simulink model "ElectricVehicleNMPC"  (R2022b)
settings: Solver=VariableStepAuto  StartTime=0  StopTime=600+N*Ts  RelTol=1e-3
model workspace (MAT data in the model file):
  AccessaryLoad = Simulink.Parameter
  AccessaryLoad.Value = 600
  AccessaryLoad.Description = 'Extra power comsumed in the vehicle.
    | E.g, radio, AC, etc.'
  AccessaryLoad.DataType = 'auto'
  AccessaryLoad.Complexity = 'real'
  AccessaryLoad.Dimensions = [1 1]
  BrakeRegenFraction = Simulink.Parameter
  BrakeRegenFraction.Value = 0.55
  BrakeRegenFraction.DataType = 'auto'
  BrakeRegenFraction.Complexity = 'real'
  BrakeRegenFraction.Dimensions = [1 1]
  Crr = Simulink.Parameter
  Crr.Value = 0.01
  Crr.Description = 'Coefficient of rolling resistence
    | '
  Crr.DataType = 'auto'
  Crr.Complexity = 'real'
  Crr.Dimensions = [1 1]
  DrivelineModelG = Simulink.Parameter
  DrivelineModelG.Value = 3.55
  DrivelineModelG.DataType = 'auto'
  DrivelineModelG.Complexity = 'real'
  DrivelineModelG.Dimensions = [1 1]
  DrivelineModelSpinLoss = Simulink.Parameter
  DrivelineModelSpinLoss.Value = 6
  DrivelineModelSpinLoss.DataType = 'auto'
  DrivelineModelSpinLoss.Complexity = 'real'
  DrivelineModelSpinLoss.Dimensions = [1 1]
  EnergyCapacity = Simulink.Parameter
  EnergyCapacity.Value = 12.6
  EnergyCapacity.Description = 'Energy Capacity of the battery [kWh]'
  EnergyCapacity.DataType = 'auto'
  EnergyCapacity.Complexity = 'real'
  EnergyCapacity.Dimensions = [1 1]
  MassVehInertia = Simulink.Parameter
  MassVehInertia.Value = 2392
  MassVehInertia.Description = 'Inertia of the Vehicle
    | '
  MassVehInertia.DataType = 'auto'
  MassVehInertia.Complexity = 'real'
  MassVehInertia.Dimensions = [1 1]
  MaxPowerOutput = Simulink.Parameter
  MaxPowerOutput.Value = 100000
  MaxPowerOutput.DataType = 'auto'
  MaxPowerOutput.Complexity = 'real'
  MaxPowerOutput.Dimensions = [1 1]
  MaxTorqueOutput = Simulink.Parameter
  MaxTorqueOutput.Value = 500
  MaxTorqueOutput.DataType = 'auto'
  MaxTorqueOutput.Complexity = 'real'
  MaxTorqueOutput.Dimensions = [1 1]
  MaximumBreakForce = Simulink.Parameter
  MaximumBreakForce.Value = 10000
  MaximumBreakForce.Description = 'Maximum Break Force [N]'
  MaximumBreakForce.DataType = 'auto'
  MaximumBreakForce.Complexity = 'real'
  MaximumBreakForce.Dimensions = [1 1]
  MotorModelC = Simulink.Parameter
  MotorModelC.Value = 628.2974
  MotorModelC.DataType = 'auto'
  MotorModelC.Complexity = 'real'
  MotorModelC.Dimensions = [1 1]
  MotorModelKc = Simulink.Parameter
  MotorModelKc.Value = 0.045237
  MotorModelKc.DataType = 'auto'
  MotorModelKc.Complexity = 'real'
  MotorModelKc.Dimensions = [1 1]
  MotorModelKi = Simulink.Parameter
  MotorModelKi.Value = 0.0167
  MotorModelKi.DataType = 'auto'
  MotorModelKi.Complexity = 'real'
  MotorModelKi.Dimensions = [1 1]
  MotorModelKw = Simulink.Parameter
  MotorModelKw.Value = 5.06640055941e-05
  MotorModelKw.DataType = 'auto'
  MotorModelKw.Complexity = 'real'
  MotorModelKw.Dimensions = [1 1]
  N = Simulink.Parameter
  N.Value = 10
  N.Description = 'The number of reference preview for NMPC
    | '
  N.DataType = 'auto'
  N.Complexity = 'real'
  N.Dimensions = [1 1]
  Q = Simulink.Parameter
  Q.Value = 100
  Q.Description = 'Weighting factor of velocity error for cost function
    | '
  Q.DataType = 'auto'
  Q.Complexity = 'real'
  Q.Dimensions = [1 1]
  Rint = Simulink.Parameter
  Rint.Value = 0.1
  Rint.Description = 'Internal Resistence of the battery
    | '
  Rint.DataType = 'auto'
  Rint.Complexity = 'real'
  Rint.Dimensions = [1 1]
  Ts = Simulink.Parameter
  Ts.Value = 0.01
  Ts.Description = 'Sample Time'
  Ts.DataType = 'auto'
  Ts.Complexity = 'real'
  Ts.Dimensions = [1 1]
  Voc = Simulink.Parameter
  Voc.Value = 340
  Voc.Description = 'Open Circuit Voltage of the Battery'
  Voc.DataType = 'auto'
  Voc.Complexity = 'real'
  Voc.Dimensions = [1 1]
  gravity = Simulink.Parameter
  gravity.Value = 9.81
  gravity.Description = 'Gravity constant
    | '
  gravity.DataType = 'auto'
  gravity.Complexity = 'real'
  gravity.Dimensions = [1 1]
  massVeh = Simulink.Parameter
  massVeh.Value = 2300
  massVeh.Description = 'Vehicle Mass
    | '
  massVeh.DataType = 'auto'
  massVeh.DocUnits = 'kg'
  massVeh.Complexity = 'real'
  massVeh.Dimensions = [1 1]
  theta = Simulink.Parameter
  theta.Value = 0
  theta.Description = 'Road Grade
    | '
  theta.DataType = 'auto'
  theta.DocUnits = 'radian'
  theta.Complexity = 'real'
  theta.Dimensions = [1 1]
  wheelRadius = Simulink.Parameter
  wheelRadius.Value = 0.34
  wheelRadius.Description = 'meter'
  wheelRadius.DataType = 'auto'
  wheelRadius.Complexity = 'real'
  wheelRadius.Dimensions = [1 1]
values from neighbouring files (symbols this model uses):
  AccessaryLoad = 600    [NMPC_EV.m]
  BrakeRegenFraction = 0.55    [NMPC_EV.m]
  Crr = 0.01    [NMPC_EV.m]
  DrivelineModelG = 3.55    [NMPC_EV.m]
  DrivelineModelSpinLoss = 6    [NMPC_EV.m]
  EnergyCapacity = 12.6    [NMPC_EV.m]
  gravity = 9.81    [NMPC_EV.m]
  m = 2    [NMPC_EV.m]
  massVeh = 2300    [NMPC_EV.m]
  MassVehInertia = 2392    [NMPC_EV.m]
  MaximumBreakForce = 10000    [NMPC_EV.m]
  MaxPowerOutput = 1e5    (= 100000)    [NMPC_EV.m]
  MaxTorqueOutput = 500    [NMPC_EV.m]
  MotorModelC = 628.2974    [NMPC_EV.m]
  MotorModelKc = 0.045237    [NMPC_EV.m]
  MotorModelKi = 0.0167    [NMPC_EV.m]
  MotorModelKw = 5.06640055940796E-5    (= 5.06640055941e-05)    [NMPC_EV.m]
  N = 5    [NMPC_EV.m]
  Q = 3000    [NMPC_EV.m]
  Rint = 0.1    [NMPC_EV.m]
  Ts = 0.01    [NMPC_EV.m]
  Voc = 340    [NMPC_EV.m]
  wheelRadius = 0.34    [NMPC_EV.m]
libraries: simulink x12, autolibshared x2
(part 1 of 2)
settings Model: SimulationMode=accelerator  Creator=allen  LastModifiedBy=allen

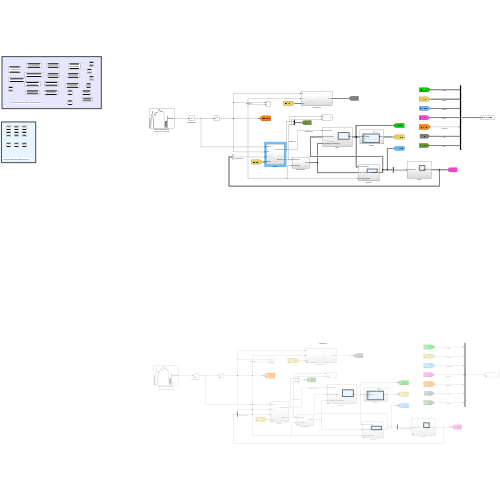
[thumbnail: Simulink's stored preview of the top-level diagram]
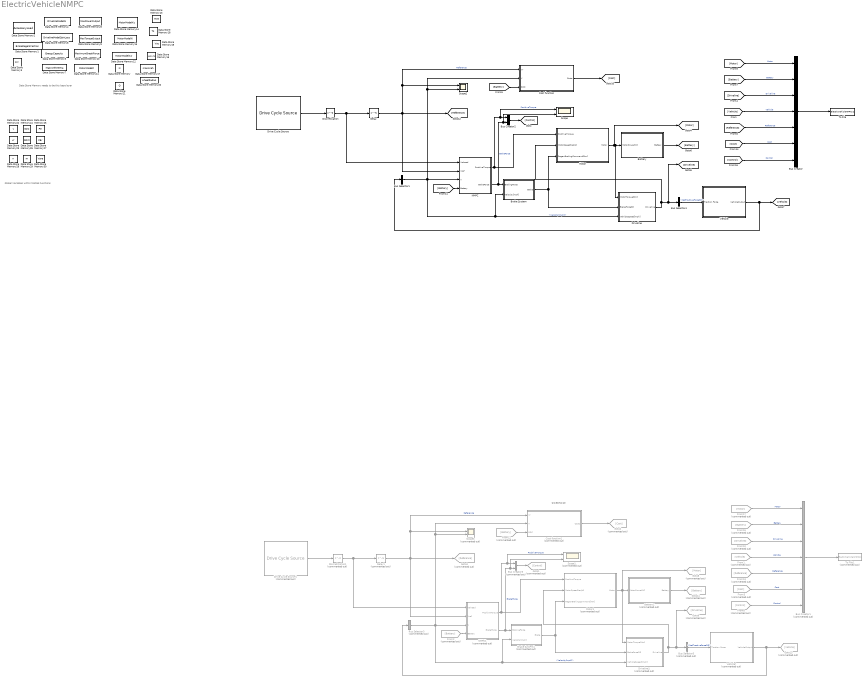
== system ElectricVehicleNMPC ==
  note: Q=30;N=10
  note: Global Variables within Matlab Functions
  note: Data Store Memory needs to be this base layer
  Battery : Subsystem
  Battery1 : Subsystem  Commented=on
  Brake System : Subsystem
  Brake System1 : Subsystem  Commented=on
  Bus Creator : BusCreator  Inputs=7
  Bus Creator1 : BusCreator  Commented=on  Inputs=7
  Bus Creator2 : BusCreator  Inputs=2
  Bus Creator3 : BusCreator  Commented=on  Inputs=2
  Bus Selector1 : BusSelector  OutputSignals=Velocity[mph]
  Bus Selector3 : BusSelector  Commented=on  OutputSignals=Velocity[mph]
  Bus Selector4 : BusSelector  OutputSignals=NetTractiveForce[N]
  Bus Selector5 : BusSelector  Commented=on  OutputSignals=NetTractiveForce[N]
  Cost function : Subsystem
  Cost function1 : Subsystem  Commented=on
  Data Store Memory : DataStoreMemory  DataStoreName=N  WriteAfterWriteMsg=warning  InitialValue=N  ShowAdditionalParam=off  OutDataTypeStr=double
  Data Store Memory1 : DataStoreMemory  DataStoreName=BrakeRegenFraction  WriteAfterWriteMsg=warning  InitialValue=BrakeRegenFraction  ShowAdditionalParam=off  OutDataTypeStr=double
  Data Store Memory10 : DataStoreMemory  DataStoreName=MaximumBreakForce  WriteAfterWriteMsg=warning  InitialValue=MaximumBreakForce  ShowAdditionalParam=off  OutDataTypeStr=double
  Data Store Memory11 : DataStoreMemory  DataStoreName=MotorModelC  WriteAfterWriteMsg=warning  InitialValue=MotorModelC  ShowAdditionalParam=off  OutDataTypeStr=double
  Data Store Memory12 : DataStoreMemory  DataStoreName=MotorModelKw  WriteAfterWriteMsg=warning  InitialValue=MotorModelKw  ShowAdditionalParam=off  OutDataTypeStr=double
  Data Store Memory13 : DataStoreMemory  DataStoreName=Rint  WriteAfterWriteMsg=warning  InitialValue=Rint  ShowAdditionalParam=off  OutDataTypeStr=double
  Data Store Memory14 : DataStoreMemory  DataStoreName=MotorModelKc  WriteAfterWriteMsg=warning  InitialValue=MotorModelKc  ShowAdditionalParam=off  OutDataTypeStr=double
  Data Store Memory15 : DataStoreMemory  DataStoreName=MotorModelKi  WriteAfterWriteMsg=warning  InitialValue=MotorModelKi  ShowAdditionalParam=off  OutDataTypeStr=double
  Data Store Memory16 : DataStoreMemory  DataStoreName=gravity  WriteAfterWriteMsg=warning  InitialValue=gravity  ShowAdditionalParam=off  OutDataTypeStr=double
  Data Store Memory17 : DataStoreMemory  DataStoreName=massVeh  WriteAfterWriteMsg=warning  InitialValue=massVeh  ShowAdditionalParam=off  OutDataTypeStr=double
  Data Store Memory18 : DataStoreMemory  DataStoreName=Ts  WriteAfterWriteMsg=warning  InitialValue=Ts  ShowAdditionalParam=off  OutDataTypeStr=double
  Data Store Memory19 : DataStoreMemory  DataStoreName=Voc  WriteAfterWriteMsg=warning  InitialValue=Voc  ShowAdditionalParam=off  OutDataTypeStr=double
  Data Store Memory2 : DataStoreMemory  DataStoreName=AccessaryLoad  WriteAfterWriteMsg=warning  InitialValue=AccessaryLoad  ShowAdditionalParam=off  OutDataTypeStr=double
  Data Store Memory20 : DataStoreMemory  DataStoreName=wheelRadius  WriteAfterWriteMsg=warning  InitialValue=wheelRadius  ShowAdditionalParam=off  OutDataTypeStr=double
  Data Store Memory21 : DataStoreMemory  DataStoreName=Q  WriteAfterWriteMsg=warning  InitialValue=Q  ShowAdditionalParam=off  OutDataTypeStr=double
  Data Store Memory22 : DataStoreMemory  DataStoreName=v  WriteAfterWriteMsg=warning  ShowAdditionalParam=off  OutDataTypeStr=double
  Data Store Memory23 : DataStoreMemory  DataStoreName=vr  WriteAfterWriteMsg=warning  ShowAdditionalParam=off  OutDataTypeStr=double
  Data Store Memory24 : DataStoreMemory  DataStoreName=SOC  WriteAfterWriteMsg=warning  ShowAdditionalParam=off  OutDataTypeStr=double
  Data Store Memory25 : DataStoreMemory  DataStoreName=Ptr  WriteAfterWriteMsg=warning  ShowAdditionalParam=off  OutDataTypeStr=double  Dimensions=[N+1,1]
  Data Store Memory26 : DataStoreMemory  DataStoreName=SOCr  WriteAfterWriteMsg=warning  InitialValue=100  ShowAdditionalParam=off  OutDataTypeStr=double
  Data Store Memory27 : DataStoreMemory  DataStoreName=FBr  WriteAfterWriteMsg=warning  ShowAdditionalParam=off  OutDataTypeStr=double  Dimensions=[N+1,1]
  Data Store Memory28 : DataStoreMemory  DataStoreName=n  WriteAfterWriteMsg=warning  InitialValue=2  ShowAdditionalParam=off  OutDataTypeStr=double
  Data Store Memory29 : DataStoreMemory  DataStoreName=m  WriteAfterWriteMsg=warning  InitialValue=2  ShowAdditionalParam=off  OutDataTypeStr=double
  Data Store Memory3 : DataStoreMemory  DataStoreName=Crr  WriteAfterWriteMsg=warning  InitialValue=Crr  ShowAdditionalParam=off  OutDataTypeStr=double
  Data Store Memory30 : DataStoreMemory  DataStoreName=Vpre  WriteAfterWriteMsg=warning  ShowAdditionalParam=off  OutDataTypeStr=double  Dimensions=[N+1,1]
  Data Store Memory4 : DataStoreMemory  DataStoreName=DrivelineModelG  WriteAfterWriteMsg=warning  InitialValue=DrivelineModelG  ShowAdditionalParam=off  OutDataTypeStr=double
  Data Store Memory5 : DataStoreMemory  DataStoreName=EnergyCapacity  WriteAfterWriteMsg=warning  InitialValue=EnergyCapacity  ShowAdditionalParam=off  OutDataTypeStr=double
  Data Store Memory6 : DataStoreMemory  DataStoreName=DrivelineModelSpinLoss  WriteAfterWriteMsg=warning  InitialValue=DrivelineModelSpinLoss  ShowAdditionalParam=off  OutDataTypeStr=double
  Data Store Memory7 : DataStoreMemory  DataStoreName=MassVehInertia  WriteAfterWriteMsg=warning  InitialValue=MassVehInertia  ShowAdditionalParam=off  OutDataTypeStr=double
  Data Store Memory8 : DataStoreMemory  DataStoreName=MaxPowerOutput  WriteAfterWriteMsg=warning  InitialValue=MaxPowerOutput  ShowAdditionalParam=off  OutDataTypeStr=double
  Data Store Memory9 : DataStoreMemory  DataStoreName=MaxTorqueOutput  WriteAfterWriteMsg=warning  InitialValue=MaxTorqueOutput  ShowAdditionalParam=off  OutDataTypeStr=double
  Delay : Delay  DelayLength=N
  Delay1 : Delay  Commented=on  DelayLength=N
  Discretization : Delay  DelayLength=0  SampleTime=Ts
  Discretization1 : Delay  Commented=on  DelayLength=0  SampleTime=Ts
  Drive Cycle Source : autolibshared/Drive Cycle Source  cycleVar=US06  fileVar=cycleFTP75.mat  tfinal="600  seconds"  cycleRepeat=off  outAccPort=off  outGearPort=off  gearList=No gear data  t_wot1=5  xdot_woto=0  xdot_wot1=30  t_wot2=20  xdot_wot2=0  t_wotend=30  srcUnit=m/s  outUnit=mph  srcAccUnit=m/s/s  outAccUnit=m/s^2  dt=0  aMode=1  faultOption=off  velBnd=2  velBndUnit=mph  inUnit=m/s  timeBnd=1  failOption=off  stopSim=off  maxFaultCnt=10  maxFaultTime=2  maxTotFaultTime=15  traceOption=off  dtTrace=1  traceWindow=10  lastDCname=US06  lastOutUnit=mph  lastDT=0  lastTB=1  lastSB=2  forceCalcBound=off
  Drive Cycle Source1 : autolibshared/Drive Cycle Source  Commented=on  cycleVar=US06  fileVar=cycleFTP75.mat  tfinal="600  seconds"  cycleRepeat=off  outAccPort=off  outGearPort=off  gearList=No gear data  t_wot1=5  xdot_woto=0  xdot_wot1=30  t_wot2=20  xdot_wot2=0  t_wotend=30  srcUnit=m/s  outUnit=mph  srcAccUnit=m/s/s  outAccUnit=m/s^2  dt=0  aMode=1  faultOption=off  velBnd=2  velBndUnit=mph  inUnit=m/s  timeBnd=1  failOption=off  stopSim=off  maxFaultCnt=10  maxFaultTime=2  maxTotFaultTime=15  traceOption=off  dtTrace=1  traceWindow=10  lastDCname=US06  lastOutUnit=mph  lastDT=0  lastTB=1  lastSB=2  forceCalcBound=off
  Driveline : Subsystem
  Driveline1 : Subsystem  Commented=on
  From1 : From  Commented=on  GotoTag=Vehicle
  From10 : From  Commented=on  GotoTag=Driveline
  From12 : From  Commented=on  GotoTag=Battery
  From13 : From  Commented=on  GotoTag=Reference
  From15 : From  Commented=on  GotoTag=Battery
  From17 : From  Commented=on  GotoTag=Motor
  From2 : From  Commented=on  GotoTag=Battery
  From3 : From  Commented=on  GotoTag=Cost
  From8 : From  Commented=on  GotoTag=Control
  Goto1 : Goto  Commented=on  GotoTag=Control
  Goto11 : Goto  Commented=on  GotoTag=Battery
  Goto13 : Goto  Commented=on  GotoTag=Vehicle
  Goto2 : Goto  Commented=on  GotoTag=Cost
  Goto3 : Goto  Commented=on  GotoTag=Reference
  Goto8 : Goto  Commented=on  GotoTag=Motor
  Goto9 : Goto  Commented=on  GotoTag=Driveline
  Motor : Subsystem
  Motor1 : Subsystem  Commented=on
  NMPC : Subsystem
  NMPC1 : Subsystem  Commented=on
  Scope : Scope  NumInputPorts=2
  Scope1 : Scope  Commented=on  NumInputPorts=2
  Scope2 : Scope  NumInputPorts=2
  Scope3 : Scope  Commented=on  NumInputPorts=2
  To File : ToFile  Filename=ElectricVehicleNMPCv2  MatrixName=Data  SaveFormat=Timeseries
  To File1 : ToFile  Commented=on  Filename=ElectricVehicleNMPC1k  MatrixName=Data  SaveFormat=Timeseries
  Vehicle : Subsystem
  Vehicle1 : Subsystem  Commented=on
  wires:
  Motor/1(Motor) -> [Motor], Driveline/1(MotorTorque[Nm]), Battery/1(MotorPower[W])
  Bus Selector1/1 -> Brake System/2(Velocity[mph]), Driveline/3(VehicleSpeed[mph]), Scope2/2, Cost function/2(V), NMPC/3(V)  "<Velocity[mph]>"
  Driveline/1(Driveline) -> Motor/2(MotorSpeed[rad/s]), [Driveline], Bus Selector4/1
  Drive Cycle Source/1 -> Discretization/1
  Bus Selector4/1 -> Vehicle/1(Traction Force)  "<NetTractiveForce[N]>"
  Battery/1(Battery) -> [Battery]
  Vehicle/1(VehicleOutput) -> [Vehicle], Bus Selector1/1
  [Battery] -> Cost function/3(SOC)
  Brake System/1(Brake) -> Motor/3(RegenBrakingCommand[Nm]), Driveline/2(BrakeForce[N])
  NMPC/1(PositiveTorque) -> Scope/1, Bus Creator2/1, Motor/1(PositiveTorque)  "PositiveTorque"
  NMPC/2(BrakeForce) -> Scope/2, Bus Creator2/2, Brake System/1(BrakingForce)  "BrakeForce"
  [Battery] -> NMPC/4(Battery)
  Delay/1 -> [Reference], NMPC/2(Vref), Scope2/1, Cost function/1(Vr)  "Reference"
  Discretization/1 -> NMPC/1(Vahead), Delay/1
  Bus Creator/1 -> To File/1
  [Driveline] -> Bus Creator/3  "Driveline"
  [Reference] -> Bus Creator/5  "Reference"
  [Cost] -> Bus Creator/6  "Cost"
  [Vehicle] -> Bus Creator/4  "Vehicle"
  [Motor] -> Bus Creator/1  "Motor"
  [Battery] -> Bus Creator/2  "Battery"
  Cost function/1(Costs) -> [Cost]
  Bus Creator2/1 -> [Control]
  [Control] -> Bus Creator/7  "Control"
  Battery1/1(Battery) -> Goto11/1
  Driveline1/1(Driveline) -> Motor1/2(MotorSpeed[rad/s]), Goto9/1, Bus Selector5/1
  Bus Selector5/1 -> Vehicle1/1(Traction Force)  "<NetTractiveForce[N]>"
  Delay1/1 -> Goto3/1, NMPC1/2(Vref), Scope3/1, Cost function1/1(Vr)  "Reference"
  From8/1 -> Bus Creator1/7  "Control"
  NMPC1/1(PositiveTorque) -> Scope1/1, Bus Creator3/1, Motor1/1(PositiveTorque)  "PositiveTorque"
  From1/1 -> Bus Creator1/4  "Vehicle"
  Bus Creator3/1 -> Goto1/1
  From15/1 -> Bus Creator1/2  "Battery"
  Bus Selector3/1 -> Brake System1/2(Velocity[mph]), Driveline1/3(VehicleSpeed[mph]), Scope3/2, Cost function1/2(V), NMPC1/3(V)  "<Velocity[mph]>"
  From12/1 -> Cost function1/3(SOC)
  NMPC1/2(BrakeForce) -> Scope1/2, Bus Creator3/2, Brake System1/1(BrakingForce)  "BrakeForce"
  From2/1 -> NMPC1/4(Battery)
  Discretization1/1 -> NMPC1/1(Vahead), Delay1/1
  From13/1 -> Bus Creator1/5  "Reference"
  From3/1 -> Bus Creator1/6  "Cost"
  Bus Creator1/1 -> To File1/1
  From10/1 -> Bus Creator1/3  "Driveline"
  Cost function1/1(Costs) -> Goto2/1
  Vehicle1/1(VehicleOutput) -> Goto13/1, Bus Selector3/1
  From17/1 -> Bus Creator1/1  "Motor"
  Motor1/1(Motor) -> Goto8/1, Driveline1/1(MotorTorque[Nm]), Battery1/1(MotorPower[W])
  Drive Cycle Source1/1 -> Discretization1/1
  Brake System1/1(Brake) -> Motor1/3(RegenBrakingCommand[Nm]), Driveline1/2(BrakeForce[N])

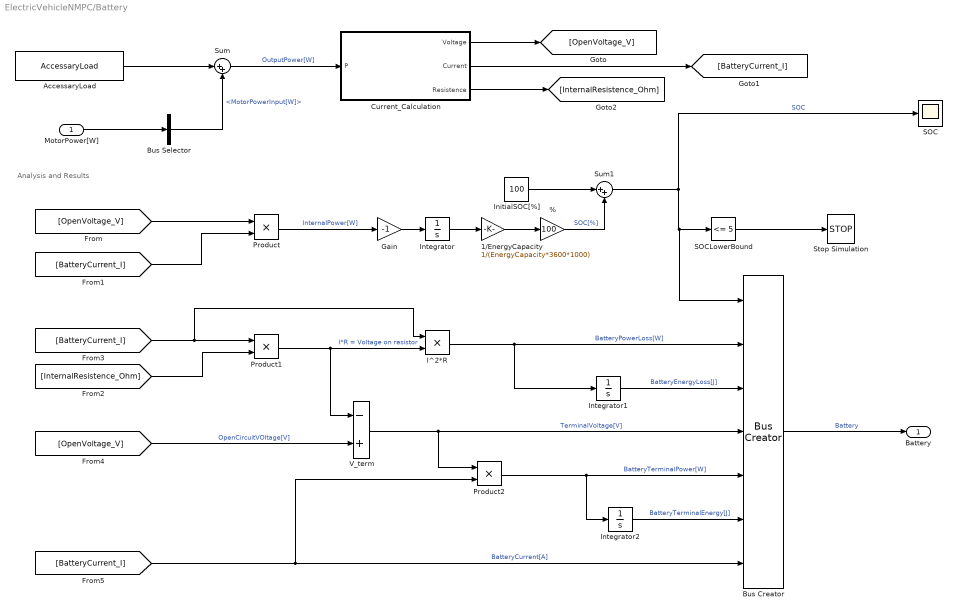
== system ElectricVehicleNMPC/Battery ==
  note: Analysis and Results
  MotorPower[W] : Inport
  % : Gain  Gain=100
  1/EnergyCapacity : Gain  Gain=1/(EnergyCapacity*3600*1000)
  AccessaryLoad : Constant  Value=AccessaryLoad
  Bus Creator : BusCreator  Inputs=7
  Bus Selector : BusSelector  OutputSignals=MotorPowerInput[W]
  Current_Calculation : Subsystem
  Gain : Gain  Gain=-1
  I^2*R : Product
  InitialSOC[%] : Constant  Value=100
  Integrator : Integrator
  Integrator1 : Integrator
  Integrator2 : Integrator
  Product : Product
  Product1 : Product
  Product2 : Product
  SOC : Scope
  SOCLowerBound : simulink/Logic and Bit Operations/Compare To Constant  relop=<=  const=5  OutDataTypeStr=boolean
  Stop Simulation : Stop
  Sum : Sum  Inputs=|++
  Sum1 : Sum  Inputs=|++
  V_term : Sum  Inputs=-+
  Battery : Outport
  wires:
  AccessaryLoad/1 -> Sum/1
  Sum/1 -> Current_Calculation/1(P)  "OutputPower[W]"
  MotorPower[W]/1 -> Bus Selector/1
  Current_Calculation/1(Voltage) -> [OpenVoltage_V]
  Current_Calculation/2(Current) -> [BatteryCurrent_I]
  Current_Calculation/3(Resistence) -> [InternalResistence_Ohm]
  [OpenVoltage_V] -> Product/1
  [BatteryCurrent_I] -> Product/2
  Product/1 -> Gain/1  "InternalPower[W]"
  Gain/1 -> Integrator/1
  Integrator/1 -> 1/EnergyCapacity/1
  1/EnergyCapacity/1 -> %/1
  %/1 -> Sum1/2  "SOC[%]"
  SOCLowerBound/1 -> Stop Simulation/1
  [BatteryCurrent_I] -> I^2*R/1, Product1/1
  [InternalResistence_Ohm] -> Product1/2
  Product1/1 -> V_term/1, I^2*R/2  "I*R = Voltage on resistor"
  I^2*R/1 -> Integrator1/1, Bus Creator/2  "BatteryPowerLoss[W]"
  Integrator1/1 -> Bus Creator/3  "BatteryEnergyLoss[J]"
  [OpenVoltage_V] -> V_term/2  "OpenCircuitVOltage[V]"
  V_term/1 -> Product2/1, Bus Creator/4  "TerminalVoltage[V]"
  [BatteryCurrent_I] -> Product2/2, Bus Creator/7  "BatteryCurrent[A]"
  Product2/1 -> Integrator2/1, Bus Creator/5  "BatteryTerminalPower[W]"
  Integrator2/1 -> Bus Creator/6  "BatteryTerminalEnergy[J]"
  Bus Creator/1 -> Battery/1  "Battery"
  Bus Selector/1 -> Sum/2  "<MotorPowerInput[W]>"
  InitialSOC[%]/1 -> Sum1/1
  Sum1/1 -> Bus Creator/1, SOCLowerBound/1, SOC/1  "SOC"

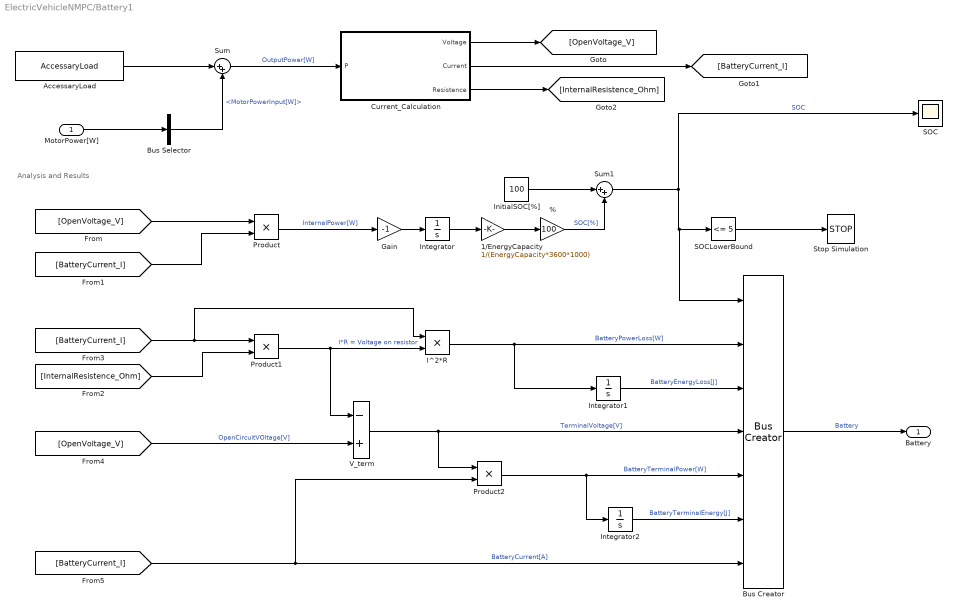
== system ElectricVehicleNMPC/Battery1 ==
  note: Analysis and Results
  MotorPower[W] : Inport
  % : Gain  Gain=100
  1/EnergyCapacity : Gain  Gain=1/(EnergyCapacity*3600*1000)
  AccessaryLoad : Constant  Value=AccessaryLoad
  Bus Creator : BusCreator  Inputs=7
  Bus Selector : BusSelector  OutputSignals=MotorPowerInput[W]
  Current_Calculation : Subsystem
  Gain : Gain  Gain=-1
  I^2*R : Product
  InitialSOC[%] : Constant  Value=100
  Integrator : Integrator
  Integrator1 : Integrator
  Integrator2 : Integrator
  Product : Product
  Product1 : Product
  Product2 : Product
  SOC : Scope
  SOCLowerBound : simulink/Logic and Bit Operations/Compare To Constant  relop=<=  const=5  OutDataTypeStr=boolean
  Stop Simulation : Stop
  Sum : Sum  Inputs=|++
  Sum1 : Sum  Inputs=|++
  V_term : Sum  Inputs=-+
  Battery : Outport
  wires:
  AccessaryLoad/1 -> Sum/1
  Sum/1 -> Current_Calculation/1(P)  "OutputPower[W]"
  MotorPower[W]/1 -> Bus Selector/1
  Current_Calculation/1(Voltage) -> [OpenVoltage_V]
  Current_Calculation/2(Current) -> [BatteryCurrent_I]
  Current_Calculation/3(Resistence) -> [InternalResistence_Ohm]
  [OpenVoltage_V] -> Product/1
  [BatteryCurrent_I] -> Product/2
  Product/1 -> Gain/1  "InternalPower[W]"
  Gain/1 -> Integrator/1
  Integrator/1 -> 1/EnergyCapacity/1
  1/EnergyCapacity/1 -> %/1
  %/1 -> Sum1/2  "SOC[%]"
  SOCLowerBound/1 -> Stop Simulation/1
  [BatteryCurrent_I] -> I^2*R/1, Product1/1
  [InternalResistence_Ohm] -> Product1/2
  Product1/1 -> V_term/1, I^2*R/2  "I*R = Voltage on resistor"
  I^2*R/1 -> Integrator1/1, Bus Creator/2  "BatteryPowerLoss[W]"
  Integrator1/1 -> Bus Creator/3  "BatteryEnergyLoss[J]"
  [OpenVoltage_V] -> V_term/2  "OpenCircuitVOltage[V]"
  V_term/1 -> Product2/1, Bus Creator/4  "TerminalVoltage[V]"
  [BatteryCurrent_I] -> Product2/2, Bus Creator/7  "BatteryCurrent[A]"
  Product2/1 -> Integrator2/1, Bus Creator/5  "BatteryTerminalPower[W]"
  Integrator2/1 -> Bus Creator/6  "BatteryTerminalEnergy[J]"
  Bus Creator/1 -> Battery/1  "Battery"
  Bus Selector/1 -> Sum/2  "<MotorPowerInput[W]>"
  InitialSOC[%]/1 -> Sum1/1
  Sum1/1 -> Bus Creator/1, SOCLowerBound/1, SOC/1  "SOC"

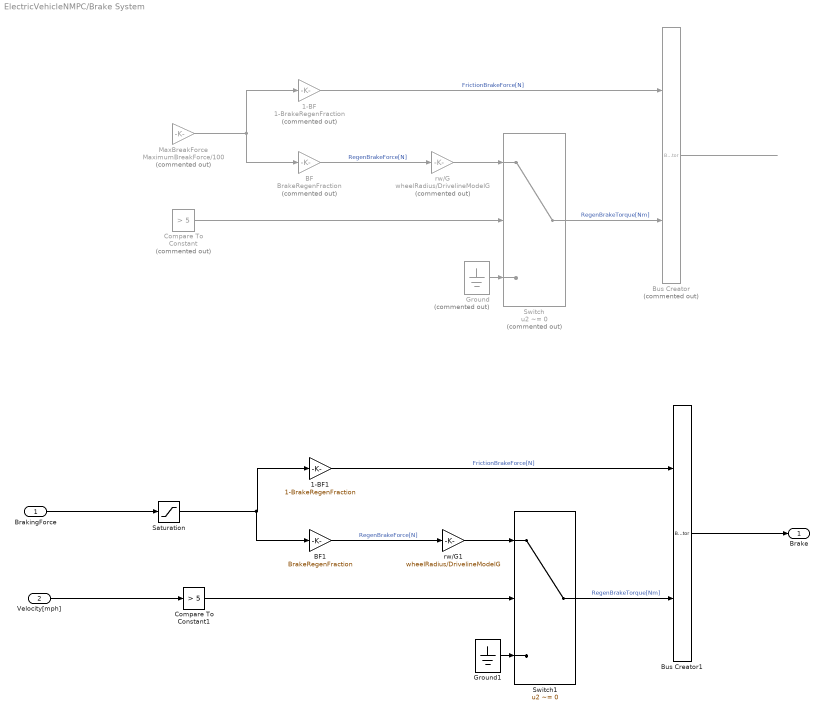
== system ElectricVehicleNMPC/Brake System ==
  BrakingForce : Inport
  Velocity[mph] : Inport  Port=2
  1-BF : Gain  Commented=on  Gain=1-BrakeRegenFraction
  1-BF1 : Gain  Gain=1-BrakeRegenFraction
  BF : Gain  Commented=on  Gain=BrakeRegenFraction
  BF1 : Gain  Gain=BrakeRegenFraction
  Bus Creator : BusCreator  Commented=on  Inputs=2
  Bus Creator1 : BusCreator  Inputs=2
  Compare To Constant : simulink/Logic and Bit Operations/Compare To Constant  Commented=on  relop=>  const=5  OutDataTypeStr=boolean
  Compare To Constant1 : simulink/Logic and Bit Operations/Compare To Constant  relop=>  const=5  OutDataTypeStr=boolean
  Ground : Ground  Commented=on
  Ground1 : Ground
  MaxBreakForce : Gain  Commented=on  Gain=MaximumBreakForce/100
  Saturation : Saturate  UpperLimit=0  LowerLimit=-MaximumBreakForce
  Switch : Switch  Commented=on  Criteria=u2 ~= 0  SaturateOnIntegerOverflow=off  InputSameDT=off
  Switch1 : Switch  Criteria=u2 ~= 0  SaturateOnIntegerOverflow=off  InputSameDT=off
  rw/G : Gain  Commented=on  Gain=wheelRadius/DrivelineModelG
  rw/G1 : Gain  Gain=wheelRadius/DrivelineModelG
  Brake : Outport
  wires:
  Compare To Constant/1 -> Switch/2
  Ground/1 -> Switch/3
  MaxBreakForce/1 -> BF/1, 1-BF/1
  BF/1 -> rw/G/1  "RegenBrakeForce[N]"
  rw/G/1 -> Switch/1
  Switch/1 -> Bus Creator/2  "RegenBrakeTorque[Nm]"
  1-BF/1 -> Bus Creator/1  "FrictionBrakeForce[N]"
  Bus Creator/1 -> ?
  Ground1/1 -> Switch1/3
  rw/G1/1 -> Switch1/1
  Switch1/1 -> Bus Creator1/2  "RegenBrakeTorque[Nm]"
  Bus Creator1/1 -> Brake/1
  Velocity[mph]/1 -> Compare To Constant1/1
  1-BF1/1 -> Bus Creator1/1  "FrictionBrakeForce[N]"
  BF1/1 -> rw/G1/1  "RegenBrakeForce[N]"
  BrakingForce/1 -> Saturation/1
  Compare To Constant1/1 -> Switch1/2
  Saturation/1 -> BF1/1, 1-BF1/1

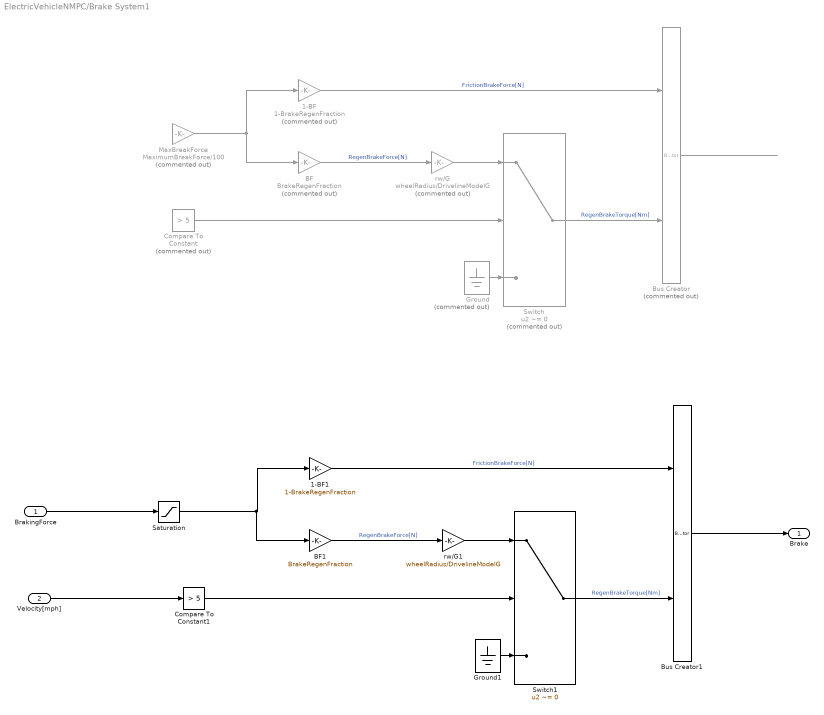
== system ElectricVehicleNMPC/Brake System1 ==
  BrakingForce : Inport
  Velocity[mph] : Inport  Port=2
  1-BF : Gain  Commented=on  Gain=1-BrakeRegenFraction
  1-BF1 : Gain  Gain=1-BrakeRegenFraction
  BF : Gain  Commented=on  Gain=BrakeRegenFraction
  BF1 : Gain  Gain=BrakeRegenFraction
  Bus Creator : BusCreator  Commented=on  Inputs=2
  Bus Creator1 : BusCreator  Inputs=2
  Compare To Constant : simulink/Logic and Bit Operations/Compare To Constant  Commented=on  relop=>  const=5  OutDataTypeStr=boolean
  Compare To Constant1 : simulink/Logic and Bit Operations/Compare To Constant  relop=>  const=5  OutDataTypeStr=boolean
  Ground : Ground  Commented=on
  Ground1 : Ground
  MaxBreakForce : Gain  Commented=on  Gain=MaximumBreakForce/100
  Saturation : Saturate  UpperLimit=0  LowerLimit=-MaximumBreakForce
  Switch : Switch  Commented=on  Criteria=u2 ~= 0  SaturateOnIntegerOverflow=off  InputSameDT=off
  Switch1 : Switch  Criteria=u2 ~= 0  SaturateOnIntegerOverflow=off  InputSameDT=off
  rw/G : Gain  Commented=on  Gain=wheelRadius/DrivelineModelG
  rw/G1 : Gain  Gain=wheelRadius/DrivelineModelG
  Brake : Outport
  wires:
  Compare To Constant/1 -> Switch/2
  Ground/1 -> Switch/3
  MaxBreakForce/1 -> BF/1, 1-BF/1
  BF/1 -> rw/G/1  "RegenBrakeForce[N]"
  rw/G/1 -> Switch/1
  Switch/1 -> Bus Creator/2  "RegenBrakeTorque[Nm]"
  1-BF/1 -> Bus Creator/1  "FrictionBrakeForce[N]"
  Bus Creator/1 -> ?
  Ground1/1 -> Switch1/3
  rw/G1/1 -> Switch1/1
  Switch1/1 -> Bus Creator1/2  "RegenBrakeTorque[Nm]"
  Bus Creator1/1 -> Brake/1
  Velocity[mph]/1 -> Compare To Constant1/1
  1-BF1/1 -> Bus Creator1/1  "FrictionBrakeForce[N]"
  BF1/1 -> rw/G1/1  "RegenBrakeForce[N]"
  BrakingForce/1 -> Saturation/1
  Compare To Constant1/1 -> Switch1/2
  Saturation/1 -> BF1/1, 1-BF1/1

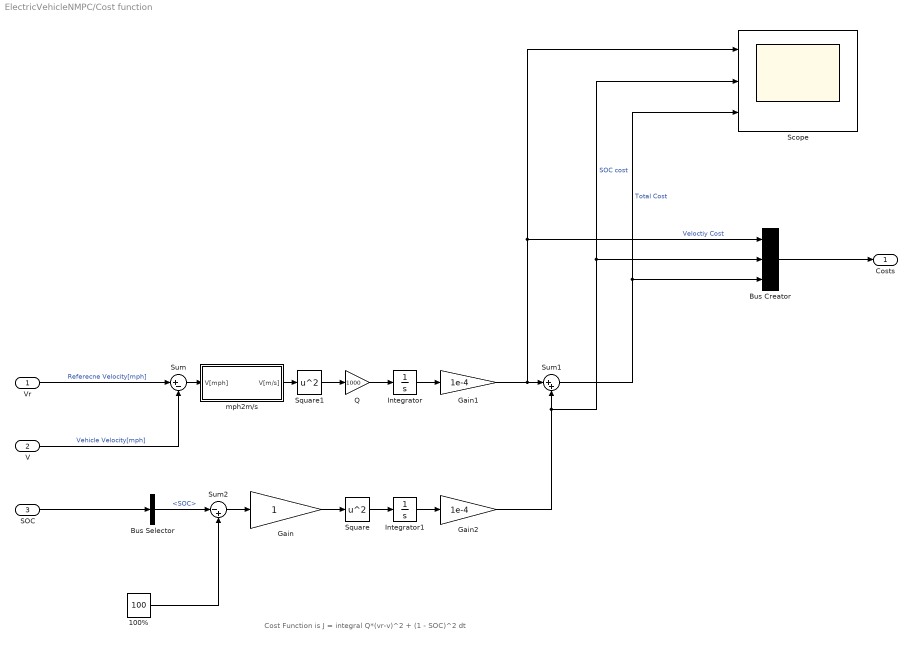
== system ElectricVehicleNMPC/Cost function ==
  note: Cost Function is J = integral Q*(vr-v)^2 + (1 - SOC)^2 dt
  Vr : Inport
  V : Inport  Port=2
  SOC : Inport  Port=3
  100% : Constant  Value=100
  Bus Creator : BusCreator  Inputs=3
  Bus Selector : BusSelector  OutputSignals=SOC
  Gain : Gain
  Gain1 : Gain  Gain=1e-4
  Gain2 : Gain  Gain=1e-4
  Integrator : Integrator
  Integrator1 : Integrator
  Q : Gain  Gain=1000
  Scope : Scope  NumInputPorts=3
  Square : Math  Operator=square
  Square1 : Math  Operator=square
  Sum : Sum  Inputs=|+-
  Sum1 : Sum  Inputs=|++
  Sum2 : Sum  Inputs=|-+
  mph2m/s : Subsystem
  Costs : Outport
  wires:
  Vr/1 -> Sum/1  "Referecne Velocity[mph]"
  V/1 -> Sum/2  "Vehicle Velocity[mph]"
  Sum/1 -> mph2m/s/1(V[mph])
  SOC/1 -> Bus Selector/1
  Sum1/1 -> Bus Creator/3, Scope/3  "Total Cost"
  Bus Selector/1 -> Sum2/1  "<SOC>"
  100%/1 -> Sum2/2
  Sum2/1 -> Gain/1
  Gain/1 -> Square/1
  Square/1 -> Integrator1/1
  Square1/1 -> Q/1
  Integrator1/1 -> Gain2/1
  Q/1 -> Integrator/1
  mph2m/s/1(V[m/s]) -> Square1/1
  Integrator/1 -> Gain1/1
  Gain2/1 -> Bus Creator/2, Scope/2, Sum1/2  "SOC cost"
  Gain1/1 -> Sum1/1, Scope/1, Bus Creator/1  "Veloctiy Cost"
  Bus Creator/1 -> Costs/1

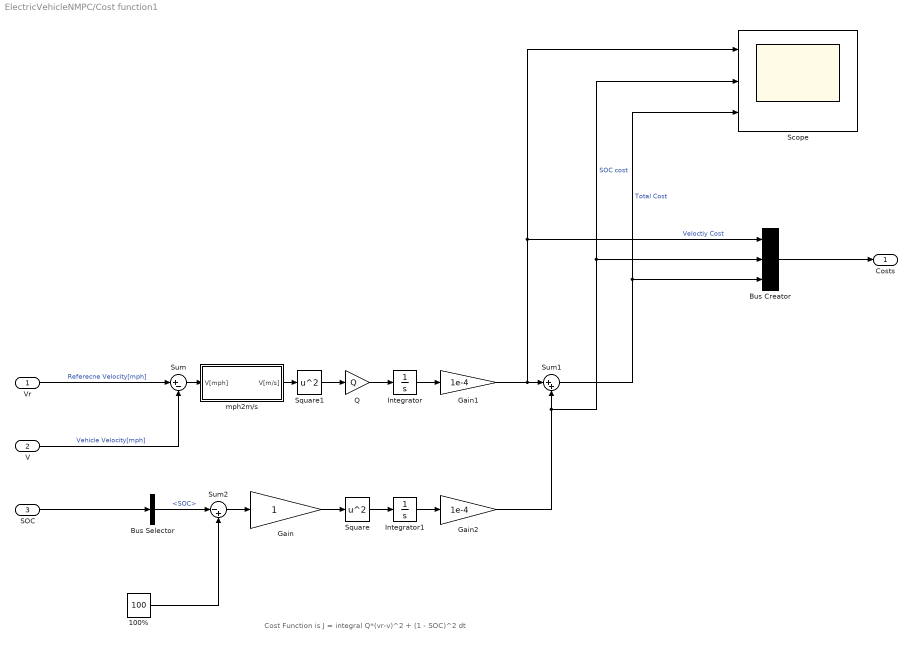
== system ElectricVehicleNMPC/Cost function1 ==
  note: Cost Function is J = integral Q*(vr-v)^2 + (1 - SOC)^2 dt
  Vr : Inport
  V : Inport  Port=2
  SOC : Inport  Port=3
  100% : Constant  Value=100
  Bus Creator : BusCreator  Inputs=3
  Bus Selector : BusSelector  OutputSignals=SOC
  Gain : Gain
  Gain1 : Gain  Gain=1e-4
  Gain2 : Gain  Gain=1e-4
  Integrator : Integrator
  Integrator1 : Integrator
  Q : Gain  Gain=Q
  Scope : Scope  NumInputPorts=3
  Square : Math  Operator=square
  Square1 : Math  Operator=square
  Sum : Sum  Inputs=|+-
  Sum1 : Sum  Inputs=|++
  Sum2 : Sum  Inputs=|-+
  mph2m/s : Subsystem
  Costs : Outport
  wires:
  Vr/1 -> Sum/1  "Referecne Velocity[mph]"
  V/1 -> Sum/2  "Vehicle Velocity[mph]"
  Sum/1 -> mph2m/s/1(V[mph])
  SOC/1 -> Bus Selector/1
  Sum1/1 -> Bus Creator/3, Scope/3  "Total Cost"
  Bus Selector/1 -> Sum2/1  "<SOC>"
  100%/1 -> Sum2/2
  Sum2/1 -> Gain/1
  Gain/1 -> Square/1
  Square/1 -> Integrator1/1
  Square1/1 -> Q/1
  Integrator1/1 -> Gain2/1
  Q/1 -> Integrator/1
  mph2m/s/1(V[m/s]) -> Square1/1
  Integrator/1 -> Gain1/1
  Gain2/1 -> Bus Creator/2, Scope/2, Sum1/2  "SOC cost"
  Gain1/1 -> Sum1/1, Scope/1, Bus Creator/1  "Veloctiy Cost"
  Bus Creator/1 -> Costs/1

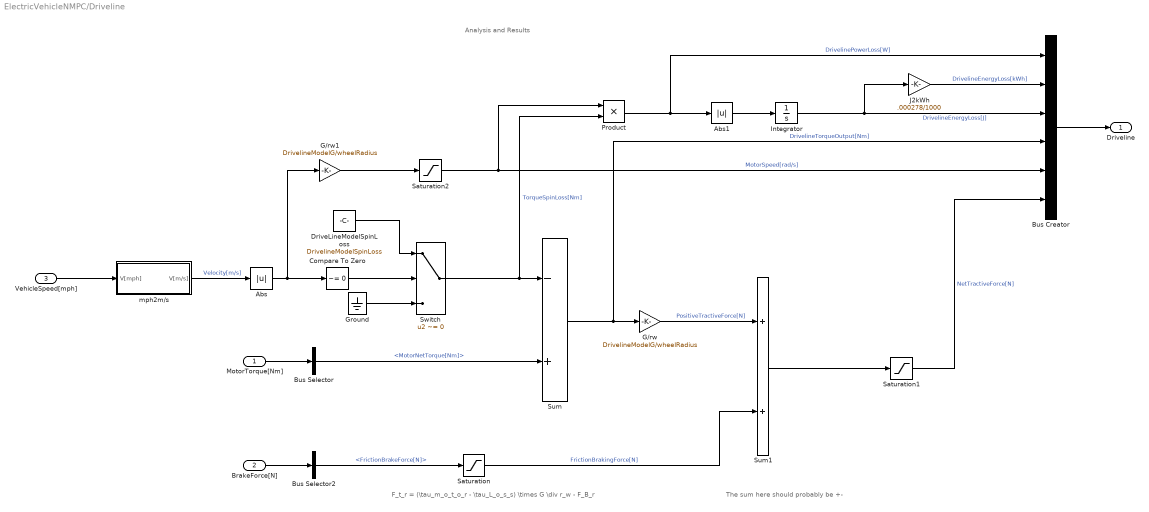
== system ElectricVehicleNMPC/Driveline ==
  note: The sum here should probably be +-
  note: F_t_r = (\tau_m_o_t_o_r - \tau_L_o_s_s) \times G \div r_w - F_B_r
  note: Analysis and Results
  MotorTorque[Nm] : Inport
  BrakeForce[N] : Inport  Port=2
  VehicleSpeed[mph] : Inport  Port=3
  Abs : Abs  SaturateOnIntegerOverflow=off
  Abs1 : Abs  SaturateOnIntegerOverflow=off
  Bus Creator : BusCreator  Inputs=6
  Bus Selector : BusSelector  OutputSignals=MotorNetTorque[Nm]
  Bus Selector2 : BusSelector  OutputSignals=FrictionBrakeForce[N]
  Compare To Zero : simulink/Logic and Bit Operations/Compare To Zero  relop=~=  OutDataTypeStr=boolean
  DriveLineModelSpinLoss : Constant  Value=DrivelineModelSpinLoss
  G/rw : Gain  Gain=DrivelineModelG/wheelRadius
  G/rw1 : Gain  Gain=DrivelineModelG/wheelRadius
  Ground : Ground
  Integrator : Integrator
  J2kWh : Gain  Gain=.000278/1000
  Product : Product
  Saturation : Saturate  UpperLimit=0  LowerLimit=-10000
  Saturation1 : Saturate  UpperLimit=5000  LowerLimit=-10000
  Saturation2 : Saturate  UpperLimit=Inf  LowerLimit=0.00001  ZeroCross=off
  Sum : Sum  Inputs=-+
  Sum1 : Sum
  Switch : Switch  Criteria=u2 ~= 0  SaturateOnIntegerOverflow=off  InputSameDT=off
  mph2m/s : Subsystem
  Driveline : Outport
  wires:
  MotorTorque[Nm]/1 -> Bus Selector/1
  Bus Selector/1 -> Sum/2  "<MotorNetTorque[Nm]>"
  VehicleSpeed[mph]/1 -> mph2m/s/1(V[mph])
  mph2m/s/1(V[m/s]) -> Abs/1  "Velocity[m/s]"
  Abs/1 -> G/rw1/1, Compare To Zero/1
  Ground/1 -> Switch/3
  Compare To Zero/1 -> Switch/2
  DriveLineModelSpinLoss/1 -> Switch/1
  Switch/1 -> Product/2, Sum/1  "TorqueSpinLoss[Nm]"
  Sum/1 -> Bus Creator/4, G/rw/1  "DrivelineTorqueOutput[Nm]"
  G/rw/1 -> Sum1/1  "PositiveTractiveForce[N]"
  Bus Selector2/1 -> Saturation/1  "<FrictionBrakeForce[N]>"
  BrakeForce[N]/1 -> Bus Selector2/1
  Saturation/1 -> Sum1/2  "FrictionBrakingForce[N]"
  Sum1/1 -> Saturation1/1
  Saturation1/1 -> Bus Creator/6  "NetTractiveForce[N]"
  G/rw1/1 -> Saturation2/1
  Saturation2/1 -> Bus Creator/5, Product/1  "MotorSpeed[rad/s]"
  Bus Creator/1 -> Driveline/1
  Product/1 -> Bus Creator/1, Abs1/1  "DrivelinePowerLoss[W]"
  Abs1/1 -> Integrator/1
  Integrator/1 -> J2kWh/1, Bus Creator/3  "DrivelineEnergyLoss[J]"
  J2kWh/1 -> Bus Creator/2  "DrivelineEnergyLoss[kWh]"

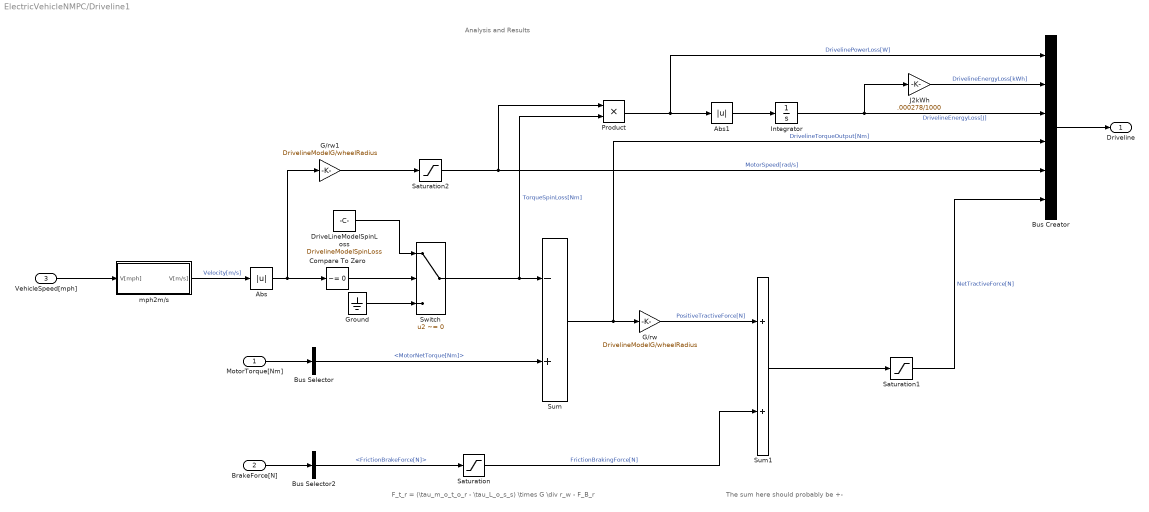
== system ElectricVehicleNMPC/Driveline1 ==
  note: The sum here should probably be +-
  note: F_t_r = (\tau_m_o_t_o_r - \tau_L_o_s_s) \times G \div r_w - F_B_r
  note: Analysis and Results
  MotorTorque[Nm] : Inport
  BrakeForce[N] : Inport  Port=2
  VehicleSpeed[mph] : Inport  Port=3
  Abs : Abs  SaturateOnIntegerOverflow=off
  Abs1 : Abs  SaturateOnIntegerOverflow=off
  Bus Creator : BusCreator  Inputs=6
  Bus Selector : BusSelector  OutputSignals=MotorNetTorque[Nm]
  Bus Selector2 : BusSelector  OutputSignals=FrictionBrakeForce[N]
  Compare To Zero : simulink/Logic and Bit Operations/Compare To Zero  relop=~=  OutDataTypeStr=boolean
  DriveLineModelSpinLoss : Constant  Value=DrivelineModelSpinLoss
  G/rw : Gain  Gain=DrivelineModelG/wheelRadius
  G/rw1 : Gain  Gain=DrivelineModelG/wheelRadius
  Ground : Ground
  Integrator : Integrator
  J2kWh : Gain  Gain=.000278/1000
  Product : Product
  Saturation : Saturate  UpperLimit=0  LowerLimit=-10000
  Saturation1 : Saturate  UpperLimit=5000  LowerLimit=-10000
  Saturation2 : Saturate  UpperLimit=Inf  LowerLimit=0.00001  ZeroCross=off
  Sum : Sum  Inputs=-+
  Sum1 : Sum
  Switch : Switch  Criteria=u2 ~= 0  SaturateOnIntegerOverflow=off  InputSameDT=off
  mph2m/s : Subsystem
  Driveline : Outport
  wires:
  MotorTorque[Nm]/1 -> Bus Selector/1
  Bus Selector/1 -> Sum/2  "<MotorNetTorque[Nm]>"
  VehicleSpeed[mph]/1 -> mph2m/s/1(V[mph])
  mph2m/s/1(V[m/s]) -> Abs/1  "Velocity[m/s]"
  Abs/1 -> G/rw1/1, Compare To Zero/1
  Ground/1 -> Switch/3
  Compare To Zero/1 -> Switch/2
  DriveLineModelSpinLoss/1 -> Switch/1
  Switch/1 -> Product/2, Sum/1  "TorqueSpinLoss[Nm]"
  Sum/1 -> Bus Creator/4, G/rw/1  "DrivelineTorqueOutput[Nm]"
  G/rw/1 -> Sum1/1  "PositiveTractiveForce[N]"
  Bus Selector2/1 -> Saturation/1  "<FrictionBrakeForce[N]>"
  BrakeForce[N]/1 -> Bus Selector2/1
  Saturation/1 -> Sum1/2  "FrictionBrakingForce[N]"
  Sum1/1 -> Saturation1/1
  Saturation1/1 -> Bus Creator/6  "NetTractiveForce[N]"
  G/rw1/1 -> Saturation2/1
  Saturation2/1 -> Bus Creator/5, Product/1  "MotorSpeed[rad/s]"
  Bus Creator/1 -> Driveline/1
  Product/1 -> Bus Creator/1, Abs1/1  "DrivelinePowerLoss[W]"
  Abs1/1 -> Integrator/1
  Integrator/1 -> J2kWh/1, Bus Creator/3  "DrivelineEnergyLoss[J]"
  J2kWh/1 -> Bus Creator/2  "DrivelineEnergyLoss[kWh]"

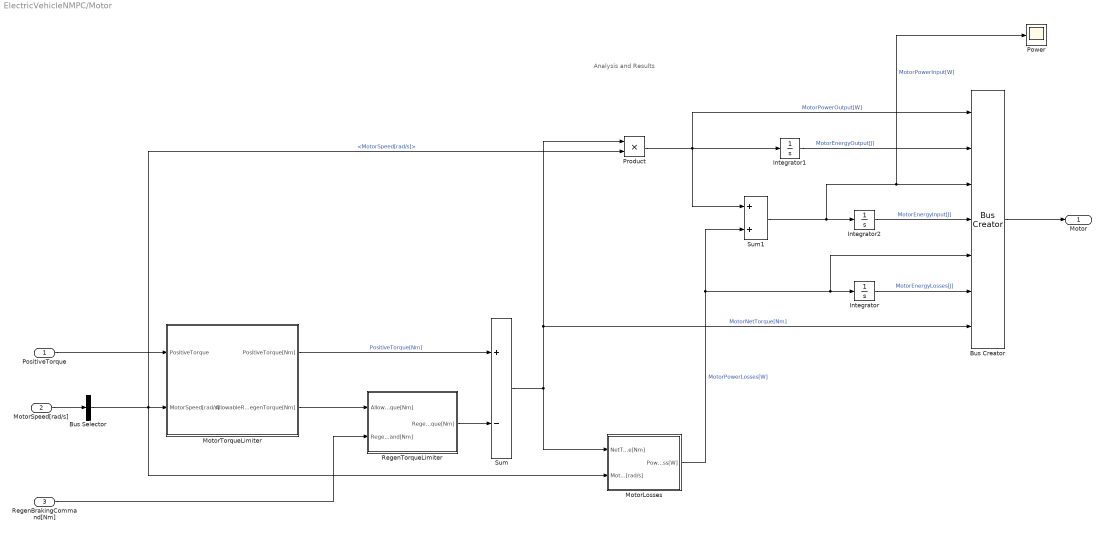
== system ElectricVehicleNMPC/Motor ==
  note: Analysis and Results
  PositiveTorque : Inport
  MotorSpeed[rad/s] : Inport  Port=2
  RegenBrakingCommand[Nm] : Inport  Port=3
  Bus Creator : BusCreator  Inputs=7
  Bus Selector : BusSelector  OutputSignals=MotorSpeed[rad/s]
  Integrator : Integrator
  Integrator1 : Integrator
  Integrator2 : Integrator
  MotorLosses : Subsystem
  MotorTorqueLimiter : Subsystem
  Power : Scope
  Product : Product
  RegenTorqueLimiter : Subsystem
  Sum : Sum  Inputs=+-
  Sum1 : Sum
  Motor : Outport
  wires:
  PositiveTorque/1 -> MotorTorqueLimiter/1(PositiveTorque)
  MotorSpeed[rad/s]/1 -> Bus Selector/1
  Bus Selector/1 -> Product/2, MotorLosses/2(MotorSpeed[rad/s]), MotorTorqueLimiter/2(MotorSpeed[rad/s])  "<MotorSpeed[rad/s]>"
  MotorTorqueLimiter/1(PositiveTorque[Nm]) -> Sum/1  "PositiveTorque[Nm]"
  MotorTorqueLimiter/2(AllowableRegenTorque[Nm]) -> RegenTorqueLimiter/1(AllowableRegenTorque[Nm])
  RegenBrakingCommand[Nm]/1 -> RegenTorqueLimiter/2(RegenBrakeCommand[Nm])
  RegenTorqueLimiter/1(RegenTorque[Nm]) -> Sum/2
  Sum/1 -> MotorLosses/1(NetTorque[Nm]), Product/1, Bus Creator/7  "MotorNetTorque[Nm]"
  Bus Creator/1 -> Motor/1
  MotorLosses/1(PowerLoss[W]) -> Bus Creator/5, Integrator/1, Sum1/2  "MotorPowerLosses[W]"
  Integrator/1 -> Bus Creator/6  "MotorEnergyLosses[J]"
  Product/1 -> Sum1/1, Integrator1/1, Bus Creator/1  "MotorPowerOutput[W]"
  Integrator1/1 -> Bus Creator/2  "MotorEnergyOutput[J]"
  Sum1/1 -> Power/1, Bus Creator/3, Integrator2/1  "MotorPowerInput[W]"
  Integrator2/1 -> Bus Creator/4  "MotorEnergyInput[J]"

== system ElectricVehicleNMPC/Motor1 ==
  note: Analysis and Results
  PositiveTorque : Inport
  MotorSpeed[rad/s] : Inport  Port=2
  RegenBrakingCommand[Nm] : Inport  Port=3
  Bus Creator : BusCreator  Inputs=7
  Bus Selector : BusSelector  OutputSignals=MotorSpeed[rad/s]
  Integrator : Integrator
  Integrator1 : Integrator
  Integrator2 : Integrator
  MotorLosses : Subsystem
  MotorTorqueLimiter : Subsystem
  Power : Scope
  Product : Product
  RegenTorqueLimiter : Subsystem
  Sum : Sum  Inputs=+-
  Sum1 : Sum
  Motor : Outport
  wires:
  PositiveTorque/1 -> MotorTorqueLimiter/1(PositiveTorque)
  MotorSpeed[rad/s]/1 -> Bus Selector/1
  Bus Selector/1 -> Product/2, MotorLosses/2(MotorSpeed[rad/s]), MotorTorqueLimiter/2(MotorSpeed[rad/s])  "<MotorSpeed[rad/s]>"
  MotorTorqueLimiter/1(PositiveTorque[Nm]) -> Sum/1  "PositiveTorque[Nm]"
  MotorTorqueLimiter/2(AllowableRegenTorque[Nm]) -> RegenTorqueLimiter/1(AllowableRegenTorque[Nm])
  RegenBrakingCommand[Nm]/1 -> RegenTorqueLimiter/2(RegenBrakeCommand[Nm])
  RegenTorqueLimiter/1(RegenTorque[Nm]) -> Sum/2
  Sum/1 -> MotorLosses/1(NetTorque[Nm]), Product/1, Bus Creator/7  "MotorNetTorque[Nm]"
  Bus Creator/1 -> Motor/1
  MotorLosses/1(PowerLoss[W]) -> Bus Creator/5, Integrator/1, Sum1/2  "MotorPowerLosses[W]"
  Integrator/1 -> Bus Creator/6  "MotorEnergyLosses[J]"
  Product/1 -> Sum1/1, Integrator1/1, Bus Creator/1  "MotorPowerOutput[W]"
  Integrator1/1 -> Bus Creator/2  "MotorEnergyOutput[J]"
  Sum1/1 -> Power/1, Bus Creator/3, Integrator2/1  "MotorPowerInput[W]"
  Integrator2/1 -> Bus Creator/4  "MotorEnergyInput[J]"

== system ElectricVehicleNMPC/NMPC ==
  Vahead : Inport
  Vref : Inport  Port=2
  V : Inport  Port=3
  Battery : Inport  Port=4
  Bus Selector : BusSelector  OutputSignals=SOC
  MATLAB Function : MATLAB Function  TreatAsAtomicUnit=on
  Zero-Order Hold : ZeroOrderHold  SampleTime=Ts
  Zero-Order Hold1 : ZeroOrderHold  SampleTime=Ts
  mph2m/s : Subsystem
  mph2m/s1 : Subsystem
  mph2m/s2 : Subsystem
  PositiveTorque : Outport
  BrakeForce : Outport  Port=2
  wires:
  Vahead/1 -> mph2m/s/1(V[mph])  "CycleVelocity[mph]"
  V/1 -> mph2m/s1/1(V[mph])  "VehicleVelocity[mph]"
  MATLAB Function/2(FB) -> Zero-Order Hold1/1
  MATLAB Function/1(Pt) -> Zero-Order Hold/1
  Battery/1 -> Bus Selector/1
  Bus Selector/1 -> MATLAB Function/4(soc)  "<SOC>"
  mph2m/s1/1(V[m/s]) -> MATLAB Function/3(VehicleV)  "Velocity[m/s]"
  mph2m/s/1(V[m/s]) -> MATLAB Function/1(Vahead)  "Velocity[m/s]"
  mph2m/s2/1(V[m/s]) -> MATLAB Function/2(Vref)  "Velocity[m/s]"
  Vref/1 -> mph2m/s2/1(V[mph])  "CycleVelocity[mph]"
  Zero-Order Hold/1 -> PositiveTorque/1
  Zero-Order Hold1/1 -> BrakeForce/1

== system ElectricVehicleNMPC/NMPC1 ==
  Vahead : Inport
  Vref : Inport  Port=2
  V : Inport  Port=3
  Battery : Inport  Port=4
  Bus Selector : BusSelector  OutputSignals=SOC
  MATLAB Function : MATLAB Function  TreatAsAtomicUnit=on
  Zero-Order Hold : ZeroOrderHold  SampleTime=Ts
  Zero-Order Hold1 : ZeroOrderHold  SampleTime=Ts
  mph2m/s : Subsystem
  mph2m/s1 : Subsystem
  mph2m/s2 : Subsystem
  PositiveTorque : Outport
  BrakeForce : Outport  Port=2
  wires:
  Vahead/1 -> mph2m/s/1(V[mph])  "CycleVelocity[mph]"
  V/1 -> mph2m/s1/1(V[mph])  "VehicleVelocity[mph]"
  MATLAB Function/2(FB) -> Zero-Order Hold1/1
  MATLAB Function/1(Pt) -> Zero-Order Hold/1
  Battery/1 -> Bus Selector/1
  Bus Selector/1 -> MATLAB Function/4(soc)  "<SOC>"
  mph2m/s1/1(V[m/s]) -> MATLAB Function/3(VehicleV)  "Velocity[m/s]"
  mph2m/s/1(V[m/s]) -> MATLAB Function/1(Vahead)  "Velocity[m/s]"
  mph2m/s2/1(V[m/s]) -> MATLAB Function/2(Vref)  "Velocity[m/s]"
  Vref/1 -> mph2m/s2/1(V[mph])  "CycleVelocity[mph]"
  Zero-Order Hold/1 -> PositiveTorque/1
  Zero-Order Hold1/1 -> BrakeForce/1

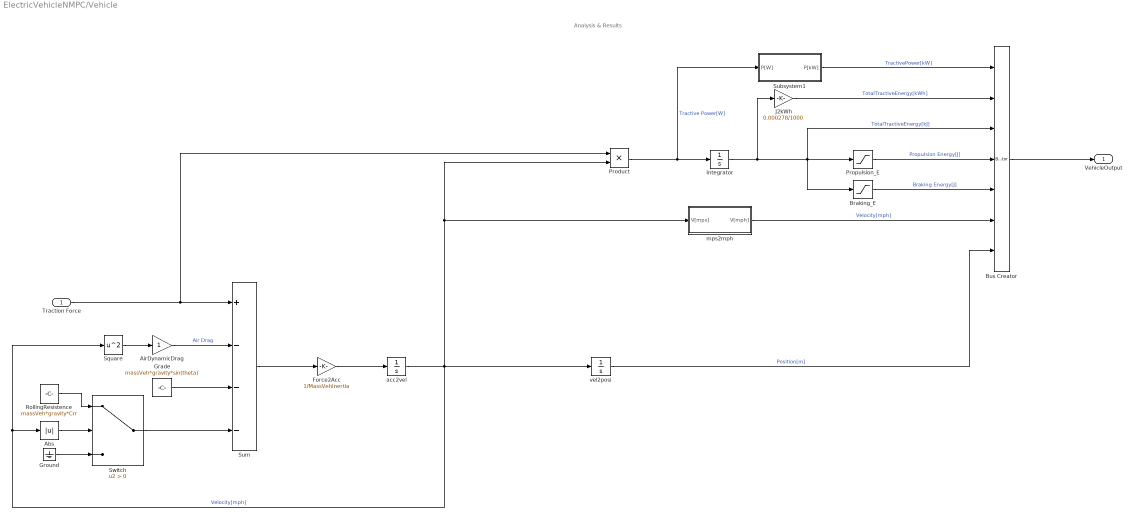
== system ElectricVehicleNMPC/Vehicle ==
  note: Analysis & Results
  Traction Force : Inport
  Abs : Abs  SaturateOnIntegerOverflow=off
  AirDynamicDrag : Gain
  Braking_E : Saturate  UpperLimit=0  LowerLimit=-Inf
  Bus Creator : BusCreator  Inputs=7
  Force2Acc : Gain  Gain=1/MassVehInertia
  Grade : Constant  Value=massVeh*gravity*sin(theta)
  Ground : Ground
  Integrator : Integrator
  J2kWh : Gain  Gain=0.000278/1000
  Product : Product
  Propulsion_E : Saturate  UpperLimit=Inf  LowerLimit=0
  RollingResistence : Constant  Value=massVeh*gravity*Crr
  Square : Math  Operator=square
  Subsystem1 : Subsystem
  Sum : Sum  Inputs=+---
  Switch : Switch  Criteria=u2 > Threshold  SaturateOnIntegerOverflow=off  InputSameDT=off
  acc2vel : Integrator
  mps2mph : Subsystem
  vel2posi : Integrator
  VehicleOutput : Outport
  wires:
  Traction Force/1 -> Product/1, Sum/1
  AirDynamicDrag/1 -> Sum/2  "Air Drag"
  Square/1 -> AirDynamicDrag/1
  Grade/1 -> Sum/3
  Switch/1 -> Sum/4
  Sum/1 -> Force2Acc/1
  Force2Acc/1 -> acc2vel/1
  acc2vel/1 -> Square/1, Abs/1, vel2posi/1, Product/2, mps2mph/1(V[mps])  "Velocity[mph]"
  vel2posi/1 -> Bus Creator/7  "Position[m]"
  Product/1 -> Integrator/1, Subsystem1/1(P[W])  "Tractive Power[W]"
  Subsystem1/1(P[kW]) -> Bus Creator/1  "TractivePower[kW]"
  J2kWh/1 -> Bus Creator/2  "TotalTractiveEnergy[kWh]"
  Propulsion_E/1 -> Bus Creator/4  "Propulsion Energy[J]"
  Braking_E/1 -> Bus Creator/5  "Braking Energy[J]"
  Integrator/1 -> Braking_E/1, Bus Creator/3, Propulsion_E/1, J2kWh/1  "TotalTractiveEnergy[kJ]"
  Bus Creator/1 -> VehicleOutput/1
  mps2mph/1(V[mph]) -> Bus Creator/6  "Velocity[mph]"
  Ground/1 -> Switch/3
  RollingResistence/1 -> Switch/1
  Abs/1 -> Switch/2

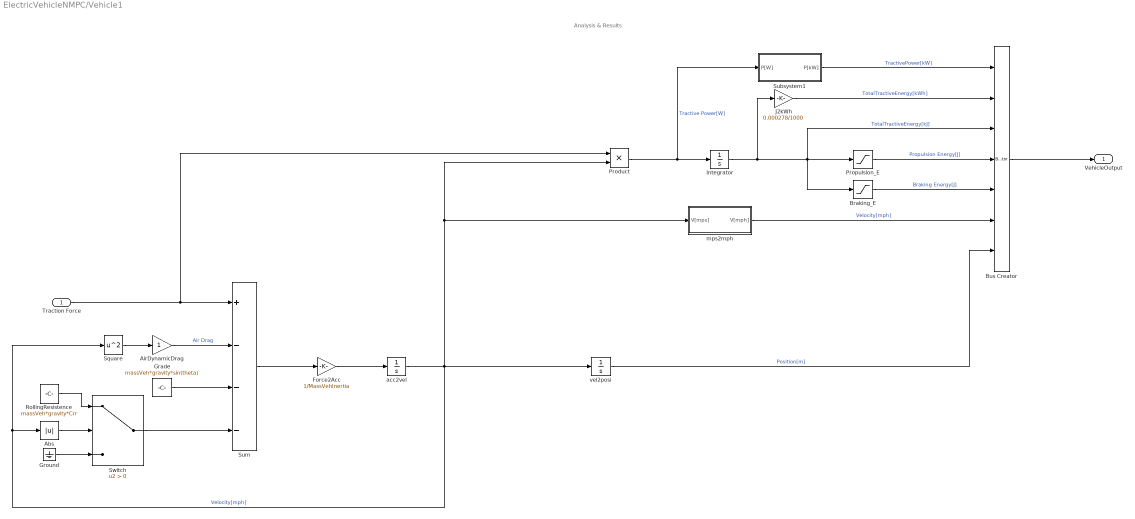
== system ElectricVehicleNMPC/Vehicle1 ==
  note: Analysis & Results
  Traction Force : Inport
  Abs : Abs  SaturateOnIntegerOverflow=off
  AirDynamicDrag : Gain
  Braking_E : Saturate  UpperLimit=0  LowerLimit=-Inf
  Bus Creator : BusCreator  Inputs=7
  Force2Acc : Gain  Gain=1/MassVehInertia
  Grade : Constant  Value=massVeh*gravity*sin(theta)
  Ground : Ground
  Integrator : Integrator
  J2kWh : Gain  Gain=0.000278/1000
  Product : Product
  Propulsion_E : Saturate  UpperLimit=Inf  LowerLimit=0
  RollingResistence : Constant  Value=massVeh*gravity*Crr
  Square : Math  Operator=square
  Subsystem1 : Subsystem
  Sum : Sum  Inputs=+---
  Switch : Switch  Criteria=u2 > Threshold  SaturateOnIntegerOverflow=off  InputSameDT=off
  acc2vel : Integrator
  mps2mph : Subsystem
  vel2posi : Integrator
  VehicleOutput : Outport
  wires:
  Traction Force/1 -> Product/1, Sum/1
  AirDynamicDrag/1 -> Sum/2  "Air Drag"
  Square/1 -> AirDynamicDrag/1
  Grade/1 -> Sum/3
  Switch/1 -> Sum/4
  Sum/1 -> Force2Acc/1
  Force2Acc/1 -> acc2vel/1
  acc2vel/1 -> Square/1, Abs/1, vel2posi/1, Product/2, mps2mph/1(V[mps])  "Velocity[mph]"
  vel2posi/1 -> Bus Creator/7  "Position[m]"
  Product/1 -> Integrator/1, Subsystem1/1(P[W])  "Tractive Power[W]"
  Subsystem1/1(P[kW]) -> Bus Creator/1  "TractivePower[kW]"
  J2kWh/1 -> Bus Creator/2  "TotalTractiveEnergy[kWh]"
  Propulsion_E/1 -> Bus Creator/4  "Propulsion Energy[J]"
  Braking_E/1 -> Bus Creator/5  "Braking Energy[J]"
  Integrator/1 -> Braking_E/1, Bus Creator/3, Propulsion_E/1, J2kWh/1  "TotalTractiveEnergy[kJ]"
  Bus Creator/1 -> VehicleOutput/1
  mps2mph/1(V[mph]) -> Bus Creator/6  "Velocity[mph]"
  Ground/1 -> Switch/3
  RollingResistence/1 -> Switch/1
  Abs/1 -> Switch/2

== system ElectricVehicleNMPC/Battery/Current_Calculation ==
  P : Inport
  Add : Sum  Inputs=+-
  Add1 : Sum  Inputs=+-
  Divide : Product  Inputs=*/
  Gain : Gain  Gain=4
  Gain1 : Gain  Gain=2
  InternalResistence : Constant  Value=Rint
  Math Function : Math  Operator=square  SignedPower=on
  OpenVoltage : Constant  Value=Voc
  Product : Product  RndMeth=Zero
  Sqrt : Sqrt
  Voltage : Outport
  Current : Outport  Port=2
  Resistence : Outport  Port=3
  wires:
  Product/1 -> Gain/1
  Divide/1 -> Current/1  "BatteryCurrent[A]"
  Math Function/1 -> Add/1
  Sqrt/1 -> Add1/2
  Gain1/1 -> Divide/2
  InternalResistence/1 -> Resistence/1, Gain1/1, Product/1  "InternalResistance[Ohm]"
  Add/1 -> Sqrt/1
  P/1 -> Product/2
  OpenVoltage/1 -> Math Function/1, Voltage/1, Add1/1  "OpenCircuitVoltage[V]"
  Gain/1 -> Add/2
  Add1/1 -> Divide/1

== system ElectricVehicleNMPC/Battery1/Current_Calculation ==
  P : Inport
  Add : Sum  Inputs=+-
  Add1 : Sum  Inputs=+-
  Divide : Product  Inputs=*/
  Gain : Gain  Gain=4
  Gain1 : Gain  Gain=2
  InternalResistence : Constant  Value=Rint
  Math Function : Math  Operator=square  SignedPower=on
  OpenVoltage : Constant  Value=Voc
  Product : Product  RndMeth=Zero
  Sqrt : Sqrt
  Voltage : Outport
  Current : Outport  Port=2
  Resistence : Outport  Port=3
  wires:
  Product/1 -> Gain/1
  Divide/1 -> Current/1  "BatteryCurrent[A]"
  Math Function/1 -> Add/1
  Sqrt/1 -> Add1/2
  Gain1/1 -> Divide/2
  InternalResistence/1 -> Resistence/1, Gain1/1, Product/1  "InternalResistance[Ohm]"
  Add/1 -> Sqrt/1
  P/1 -> Product/2
  OpenVoltage/1 -> Math Function/1, Voltage/1, Add1/1  "OpenCircuitVoltage[V]"
  Gain/1 -> Add/2
  Add1/1 -> Divide/1

== system ElectricVehicleNMPC/Cost function/mph2m//s ==
  V[mph] : Inport
  Signal Specification : SignalSpecification  Unit=m/s
  Signal Specification1 : SignalSpecification  Unit=mph
  Unit Conversion : UnitConversion
  V[m/s] : Outport
  wires:
  V[mph]/1 -> Signal Specification1/1
  Unit Conversion/1 -> Signal Specification/1
  Signal Specification/1 -> V[m/s]/1
  Signal Specification1/1 -> Unit Conversion/1

== system ElectricVehicleNMPC/Cost function1/mph2m//s ==
  V[mph] : Inport
  Signal Specification : SignalSpecification  Unit=m/s
  Signal Specification1 : SignalSpecification  Unit=mph
  Unit Conversion : UnitConversion
  V[m/s] : Outport
  wires:
  V[mph]/1 -> Signal Specification1/1
  Unit Conversion/1 -> Signal Specification/1
  Signal Specification/1 -> V[m/s]/1
  Signal Specification1/1 -> Unit Conversion/1

== system ElectricVehicleNMPC/Driveline/mph2m//s ==
  V[mph] : Inport
  Signal Specification : SignalSpecification  Unit=m/s
  Signal Specification1 : SignalSpecification  Unit=mph
  Unit Conversion : UnitConversion
  V[m/s] : Outport
  wires:
  V[mph]/1 -> Signal Specification1/1
  Unit Conversion/1 -> Signal Specification/1
  Signal Specification/1 -> V[m/s]/1
  Signal Specification1/1 -> Unit Conversion/1

== system ElectricVehicleNMPC/Driveline1/mph2m//s ==
  V[mph] : Inport
  Signal Specification : SignalSpecification  Unit=m/s
  Signal Specification1 : SignalSpecification  Unit=mph
  Unit Conversion : UnitConversion
  V[m/s] : Outport
  wires:
  V[mph]/1 -> Signal Specification1/1
  Unit Conversion/1 -> Signal Specification/1
  Signal Specification/1 -> V[m/s]/1
  Signal Specification1/1 -> Unit Conversion/1

== system ElectricVehicleNMPC/Motor/MotorLosses ==
  NetTorque[Nm] : Inport
  MotorSpeed[rad/s] : Inport  Port=2
  Compare To Zero : simulink/Logic and Bit Operations/Compare To Zero  relop=>  OutDataTypeStr=boolean
  Gain : Gain  Gain=MotorModelKc
  Ground : Ground
  Polynomial : Polyval  Coefs=[MotorModelKw,0,MotorModelKi,MotorModelC]
  Square : Math  Operator=square
  Sum : Sum
  Switch : Switch  Criteria=u2 ~= 0  SaturateOnIntegerOverflow=off  InputSameDT=off
  PowerLoss[W] : Outport
  wires:
  NetTorque[Nm]/1 -> Square/1
  Square/1 -> Gain/1
  Gain/1 -> Sum/1
  Polynomial/1 -> Sum/2
  MotorSpeed[rad/s]/1 -> Polynomial/1, Compare To Zero/1
  Compare To Zero/1 -> Switch/2
  Sum/1 -> Switch/1
  Switch/1 -> PowerLoss[W]/1
  Ground/1 -> Switch/3

== system ElectricVehicleNMPC/Motor/MotorTorqueLimiter ==
  PositiveTorque : Inport
  MotorSpeed[rad/s] : Inport  Port=2
  Divide : Product  Inputs=*/
  FractionOfMaxTorque : Gain  Gain=-0.5
  MaxPowerOutput : Constant  Value=MaxPowerOutput
  MaxTorqueOutput : Constant  Value=MaxTorqueOutput
  Min : MinMax  Inputs=2
  Min1 : MinMax  Inputs=2
  PositiveTorque[Nm] : Outport
  AllowableRegenTorque[Nm] : Outport  Port=2
  wires:
  MaxPowerOutput/1 -> Divide/1
  MotorSpeed[rad/s]/1 -> Divide/2
  MaxTorqueOutput/1 -> Min/1
  Divide/1 -> Min/2
  Min/1 -> Min1/2, FractionOfMaxTorque/1
  FractionOfMaxTorque/1 -> AllowableRegenTorque[Nm]/1  "AllowableRegenTorque[Nm]"
  PositiveTorque/1 -> Min1/1
  Min1/1 -> PositiveTorque[Nm]/1

== system ElectricVehicleNMPC/Motor/RegenTorqueLimiter ==
  AllowableRegenTorque[Nm] : Inport
  RegenBrakeCommand[Nm] : Inport  Port=2
  Abs : Abs  SaturateOnIntegerOverflow=off
  Bus Selector : BusSelector  OutputSignals=RegenBrakeTorque[Nm]
  Constant : Constant  Value=0
  Saturation Dynamic : simulink/Discontinuities/Saturation Dynamic  OutMin=[]  OutMax=[]  OutDataTypeStr=Inherit: Same as second input  OutDataType=fixdt(1, 16)  OutScaling=2^-10  DoSatur=off
  Scope : Scope
  RegenTorque[Nm] : Outport
  wires:
  Constant/1 -> Saturation Dynamic/1
  Bus Selector/1 -> Saturation Dynamic/2  "<RegenBrakeTorque[Nm]>"
  RegenBrakeCommand[Nm]/1 -> Bus Selector/1
  AllowableRegenTorque[Nm]/1 -> Saturation Dynamic/3  "AllowableRegenTorque[Nm]"
  Saturation Dynamic/1 -> Abs/1
  Abs/1 -> Scope/1, RegenTorque[Nm]/1

== system ElectricVehicleNMPC/Motor1/MotorLosses ==
  NetTorque[Nm] : Inport
  MotorSpeed[rad/s] : Inport  Port=2
  Compare To Zero : simulink/Logic and Bit Operations/Compare To Zero  relop=>  OutDataTypeStr=boolean
  Gain : Gain  Gain=MotorModelKc
  Ground : Ground
  Polynomial : Polyval  Coefs=[MotorModelKw,0,MotorModelKi,MotorModelC]
  Square : Math  Operator=square
  Sum : Sum
  Switch : Switch  Criteria=u2 ~= 0  SaturateOnIntegerOverflow=off  InputSameDT=off
  PowerLoss[W] : Outport
  wires:
  NetTorque[Nm]/1 -> Square/1
  Square/1 -> Gain/1
  Gain/1 -> Sum/1
  Polynomial/1 -> Sum/2
  MotorSpeed[rad/s]/1 -> Polynomial/1, Compare To Zero/1
  Compare To Zero/1 -> Switch/2
  Sum/1 -> Switch/1
  Switch/1 -> PowerLoss[W]/1
  Ground/1 -> Switch/3

== system ElectricVehicleNMPC/Motor1/MotorTorqueLimiter ==
  PositiveTorque : Inport
  MotorSpeed[rad/s] : Inport  Port=2
  Divide : Product  Inputs=*/
  FractionOfMaxTorque : Gain  Gain=-0.5
  MaxPowerOutput : Constant  Value=MaxPowerOutput
  MaxTorqueOutput : Constant  Value=MaxTorqueOutput
  Min : MinMax  Inputs=2
  Min1 : MinMax  Inputs=2
  PositiveTorque[Nm] : Outport
  AllowableRegenTorque[Nm] : Outport  Port=2
  wires:
  MaxPowerOutput/1 -> Divide/1
  MotorSpeed[rad/s]/1 -> Divide/2
  MaxTorqueOutput/1 -> Min/1
  Divide/1 -> Min/2
  Min/1 -> Min1/2, FractionOfMaxTorque/1
  FractionOfMaxTorque/1 -> AllowableRegenTorque[Nm]/1  "AllowableRegenTorque[Nm]"
  PositiveTorque/1 -> Min1/1
  Min1/1 -> PositiveTorque[Nm]/1

== system ElectricVehicleNMPC/Motor1/RegenTorqueLimiter ==
  AllowableRegenTorque[Nm] : Inport
  RegenBrakeCommand[Nm] : Inport  Port=2
  Abs : Abs  SaturateOnIntegerOverflow=off
  Bus Selector : BusSelector  OutputSignals=RegenBrakeTorque[Nm]
  Constant : Constant  Value=0
  Saturation Dynamic : simulink/Discontinuities/Saturation Dynamic  OutMin=[]  OutMax=[]  OutDataTypeStr=Inherit: Same as second input  OutDataType=fixdt(1, 16)  OutScaling=2^-10  DoSatur=off
  Scope : Scope
  RegenTorque[Nm] : Outport
  wires:
  Constant/1 -> Saturation Dynamic/1
  Bus Selector/1 -> Saturation Dynamic/2  "<RegenBrakeTorque[Nm]>"
  RegenBrakeCommand[Nm]/1 -> Bus Selector/1
  AllowableRegenTorque[Nm]/1 -> Saturation Dynamic/3  "AllowableRegenTorque[Nm]"
  Saturation Dynamic/1 -> Abs/1
  Abs/1 -> Scope/1, RegenTorque[Nm]/1

== system ElectricVehicleNMPC/NMPC/mph2m//s ==
  V[mph] : Inport
  Signal Specification : SignalSpecification  Unit=m/s
  Signal Specification1 : SignalSpecification  Unit=mph
  Unit Conversion : UnitConversion
  V[m/s] : Outport
  wires:
  V[mph]/1 -> Signal Specification1/1
  Unit Conversion/1 -> Signal Specification/1
  Signal Specification/1 -> V[m/s]/1
  Signal Specification1/1 -> Unit Conversion/1

== system ElectricVehicleNMPC/NMPC/mph2m//s1 ==
  V[mph] : Inport
  Signal Specification : SignalSpecification  Unit=m/s
  Signal Specification1 : SignalSpecification  Unit=mph
  Unit Conversion : UnitConversion
  V[m/s] : Outport
  wires:
  V[mph]/1 -> Signal Specification1/1
  Unit Conversion/1 -> Signal Specification/1
  Signal Specification/1 -> V[m/s]/1
  Signal Specification1/1 -> Unit Conversion/1

== system ElectricVehicleNMPC/NMPC/mph2m//s2 ==
  V[mph] : Inport
  Signal Specification : SignalSpecification  Unit=m/s
  Signal Specification1 : SignalSpecification  Unit=mph
  Unit Conversion : UnitConversion
  V[m/s] : Outport
  wires:
  V[mph]/1 -> Signal Specification1/1
  Unit Conversion/1 -> Signal Specification/1
  Signal Specification/1 -> V[m/s]/1
  Signal Specification1/1 -> Unit Conversion/1

== system ElectricVehicleNMPC/NMPC1/mph2m//s ==
  V[mph] : Inport
  Signal Specification : SignalSpecification  Unit=m/s
  Signal Specification1 : SignalSpecification  Unit=mph
  Unit Conversion : UnitConversion
  V[m/s] : Outport
  wires:
  V[mph]/1 -> Signal Specification1/1
  Unit Conversion/1 -> Signal Specification/1
  Signal Specification/1 -> V[m/s]/1
  Signal Specification1/1 -> Unit Conversion/1

== system ElectricVehicleNMPC/NMPC1/mph2m//s1 ==
  V[mph] : Inport
  Signal Specification : SignalSpecification  Unit=m/s
  Signal Specification1 : SignalSpecification  Unit=mph
  Unit Conversion : UnitConversion
  V[m/s] : Outport
  wires:
  V[mph]/1 -> Signal Specification1/1
  Unit Conversion/1 -> Signal Specification/1
  Signal Specification/1 -> V[m/s]/1
  Signal Specification1/1 -> Unit Conversion/1

== system ElectricVehicleNMPC/NMPC1/mph2m//s2 ==
  V[mph] : Inport
  Signal Specification : SignalSpecification  Unit=m/s
  Signal Specification1 : SignalSpecification  Unit=mph
  Unit Conversion : UnitConversion
  V[m/s] : Outport
  wires:
  V[mph]/1 -> Signal Specification1/1
  Unit Conversion/1 -> Signal Specification/1
  Signal Specification/1 -> V[m/s]/1
  Signal Specification1/1 -> Unit Conversion/1

== system ElectricVehicleNMPC/Vehicle/Subsystem1 ==
  P[W] : Inport
  Signal Specification : SignalSpecification  Unit=kW
  Signal Specification1 : SignalSpecification  Unit=W
  Unit Conversion : UnitConversion
  P[kW] : Outport
  wires:
  P[W]/1 -> Signal Specification1/1
  Unit Conversion/1 -> Signal Specification/1
  Signal Specification/1 -> P[kW]/1
  Signal Specification1/1 -> Unit Conversion/1

== system ElectricVehicleNMPC/Vehicle/mps2mph ==
  V[mps] : Inport
  Signal Specification : SignalSpecification  Unit=mph
  Signal Specification1 : SignalSpecification  Unit=m/s
  Unit Conversion : UnitConversion
  V[mph] : Outport
  wires:
  V[mps]/1 -> Signal Specification1/1
  Unit Conversion/1 -> Signal Specification/1
  Signal Specification/1 -> V[mph]/1
  Signal Specification1/1 -> Unit Conversion/1

== system ElectricVehicleNMPC/Vehicle1/Subsystem1 ==
  P[W] : Inport
  Signal Specification : SignalSpecification  Unit=kW
  Signal Specification1 : SignalSpecification  Unit=W
  Unit Conversion : UnitConversion
  P[kW] : Outport
  wires:
  P[W]/1 -> Signal Specification1/1
  Unit Conversion/1 -> Signal Specification/1
  Signal Specification/1 -> P[kW]/1
  Signal Specification1/1 -> Unit Conversion/1

== system ElectricVehicleNMPC/Vehicle1/mps2mph ==
  V[mps] : Inport
  Signal Specification : SignalSpecification  Unit=mph
  Signal Specification1 : SignalSpecification  Unit=m/s
  Unit Conversion : UnitConversion
  V[mph] : Outport
  wires:
  V[mps]/1 -> Signal Specification1/1
  Unit Conversion/1 -> Signal Specification/1
  Signal Specification/1 -> V[mph]/1
  Signal Specification1/1 -> Unit Conversion/1
